simulink model "FlightController"  (R2025a)
settings: Solver=VariableStepAuto  StartTime=0.0  StopTime=10.0  RelTol=1e-3
undefined symbols (not defined in the file): K, Kt, M
libraries: slpidlib x6
settings Model: Creator=pvsha  LastModifiedBy=pvsha

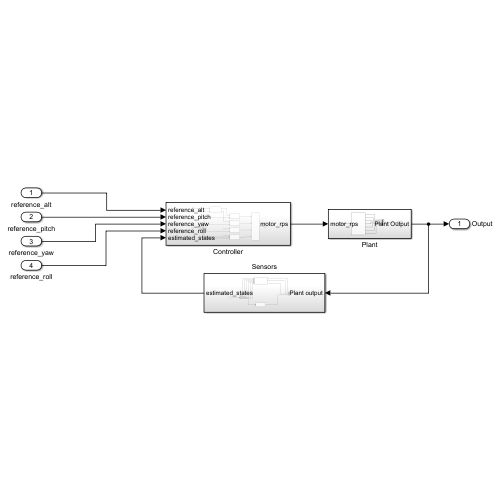
[thumbnail: Simulink's stored preview of the top-level diagram]
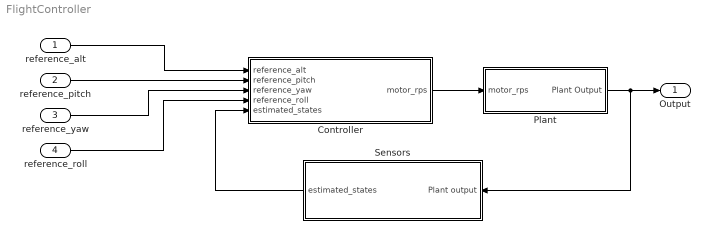
== system FlightController ==
  reference_alt : Inport
  reference_pitch : Inport  Port=2
  reference_yaw : Inport  Port=3
  reference_roll : Inport  Port=4
  Controller : Subsystem
  Plant : Subsystem
  Sensors : Subsystem
  Output : Outport  SignalName=Output
  wires:
  Controller/1(motor_rps) -> Plant/1(motor_rps)
  Sensors/1(estimated_states) -> Controller/5(estimated_states)
  Plant/1(Plant Output) -> Output/1, Sensors/1(Plant output)
  reference_alt/1 -> Controller/1(reference_alt)
  reference_pitch/1 -> Controller/2(reference_pitch)
  reference_yaw/1 -> Controller/3(reference_yaw)
  reference_roll/1 -> Controller/4(reference_roll)

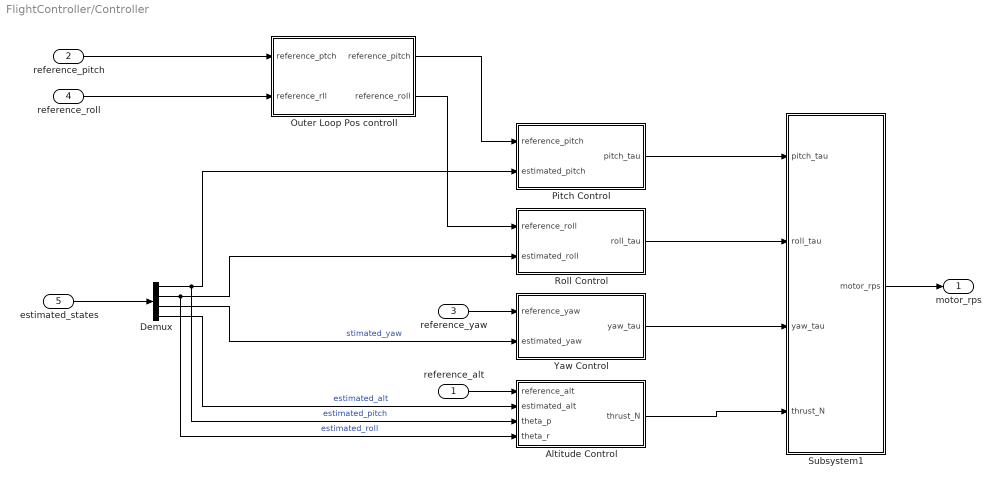
== system FlightController/Controller ==
  reference_alt : Inport
  reference_pitch : Inport  Port=2
  reference_yaw : Inport  Port=3
  reference_roll : Inport  Port=4
  estimated_states : Inport  Port=5  PortDimensions=4
  Altitude Control : Subsystem
  Demux : Demux
  Outer Loop Pos controll : Subsystem
  Pitch Control : Subsystem
  Roll Control : Subsystem
  Subsystem1 : Subsystem
  Yaw Control : Subsystem
  motor_rps : Outport
  wires:
  estimated_states/1 -> Demux/1
  Subsystem1/1(motor_rps) -> motor_rps/1
  Pitch Control/1(pitch_tau) -> Subsystem1/1(pitch_tau)
  Roll Control/1(roll_tau) -> Subsystem1/2(roll_tau)
  Altitude Control/1(thrust_N) -> Subsystem1/4(thrust_N)
  Yaw Control/1(yaw_tau) -> Subsystem1/3(yaw_tau)
  reference_yaw/1 -> Yaw Control/1(reference_yaw)
  reference_pitch/1 -> Outer Loop Pos controll/1(reference_ptch)
  reference_alt/1 -> Altitude Control/1(reference_alt)
  Demux/4 -> Altitude Control/2(estimated_alt)  "estimated_alt"
  Demux/1 -> Altitude Control/3(theta_p), Pitch Control/2(estimated_pitch)  "estimated_pitch"
  Demux/2 -> Altitude Control/4(theta_r), Roll Control/2(estimated_roll)  "estimated_roll"
  Demux/3 -> Yaw Control/2(estimated_yaw)  "stimated_yaw"
  Outer Loop Pos controll/1(reference_pitch) -> Pitch Control/1(reference_pitch)
  Outer Loop Pos controll/2(reference_roll) -> Roll Control/1(reference_roll)
  reference_roll/1 -> Outer Loop Pos controll/2(reference_rll)

== system FlightController/Plant ==
  motor_rps : Inport
  Mux : Mux  Inputs=7
  Subsystem : Subsystem
  Plant Output : Outport
  wires:
  Mux/1 -> Plant Output/1
  Subsystem/1(a_x) -> Mux/1
  Subsystem/2(a_y) -> Mux/2
  Subsystem/3(a_z) -> Mux/3
  Subsystem/4(w_p) -> Mux/4
  Subsystem/5(w_r) -> Mux/5
  Subsystem/6(w_y) -> Mux/6
  Subsystem/7(alt) -> Mux/7
  motor_rps/1 -> Subsystem/1(motor_rps)

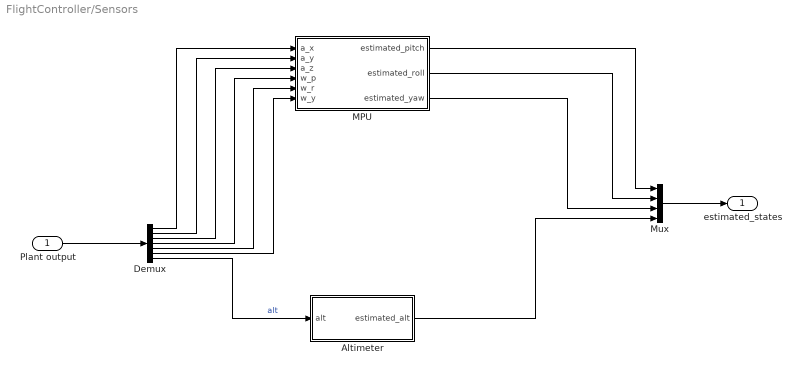
== system FlightController/Sensors ==
  Plant output : Inport
  Altimeter : Subsystem
  Demux : Demux  Outputs=7
  MPU : Subsystem
  Mux : Mux
  estimated_states : Outport
  wires:
  Plant output/1 -> Demux/1
  Demux/7 -> Altimeter/1(alt)  "alt"
  MPU/2(estimated_roll) -> Mux/2
  MPU/3(estimated_yaw) -> Mux/3
  MPU/1(estimated_pitch) -> Mux/1
  Demux/1 -> MPU/1(a_x)
  Demux/3 -> MPU/3(a_z)
  Demux/2 -> MPU/2(a_y)
  Demux/4 -> MPU/4(w_p)
  Demux/5 -> MPU/5(w_r)
  Demux/6 -> MPU/6(w_y)
  Mux/1 -> estimated_states/1
  Altimeter/1(estimated_alt) -> Mux/4

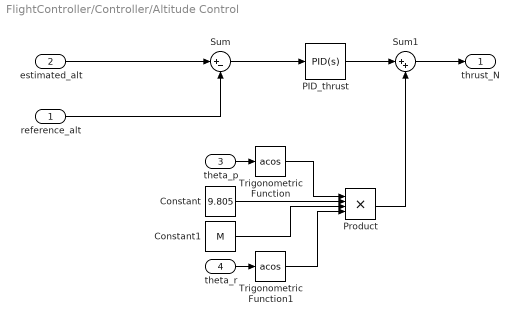
== system FlightController/Controller/Altitude Control ==
  reference_alt : Inport
  estimated_alt : Inport  Port=2
  theta_p : Inport  Port=3
  theta_r : Inport  Port=4
  Constant : Constant  Value=9.805
  Constant1 : Constant  Value=M
  PID_thrust : slpidlib/PID Controller  Controller=PID  Form=Parallel  TimeDomain=Continuous-time  UseExternalTs=off  SampleTime=-1  IntegratorMethod=Forward Euler  FilterMethod=Forward Euler  ControllerParametersSource=internal  P=1  I=1  UseKiTs=off  D=0  UseExternalDerivativeSource=off  N=100  UseFilter=on  TunerSelectOption=Transfer Function Based (PID Tuner App)  InitialConditionSource=internal  InitialConditionForIntegrator=0  InitialConditionForFilter=0  DifferentiatorICPrevScaledInput=0  ExternalReset=none  TrackingMode=off  Kt=1  LimitOutput=off  SatLimitsSource=internal  UpperSaturationLimit=inf  LowerSaturationLimit=-inf  LinearizeAsGain=on  AntiWindupMode=none  Kb=1  LimitIntegrator=off  UpperIntegratorSaturationLimit=inf  LowerIntegratorSaturationLimit=-inf  POutMin=[]  POutMax=[]  IOutMin=[]  IOutMax=[]  DOutMin=[]  DOutMax=[]  NOutMin=[]  NOutMax=[]  SumOutMin=[]  SumOutMax=[]  SaturationOutMin=[]  SaturationOutMax=[]  PParamMin=[]  PParamMax=[]  IParamMin=[]  IParamMax=[]  DParamMin=[]  DParamMax=[]  NParamMin=[]  NParamMax=[]  KbParamMin=[]  KbParamMax=[]  KtParamMin=[]  KtParamMax=[]  KbOutMin=[]  KbOutMax=[]  KtOutMin=[]  KtOutMax=[]  IntegratorOutMin=[]  IntegratorOutMax=[]  FilterOutMin=[]  FilterOutMax=[]  SumI1OutMin=[]  SumI1OutMax=[]  SumI2OutMin=[]  SumI2OutMax=[]  SumI3OutMin=[]  SumI3OutMax=[]  SumI4OutMin=[]  SumI4OutMax=[]  SumDOutMin=[]  SumDOutMax=[]  DifferentiatorOutMin=[]  DifferentiatorOutMax=[]  FilterDiffOutCoefMin=[]  FilterDiffOutCoefMax=[]  ReciprocalOutMin=[]  ReciprocalOutMax=[]  SumDenOutMin=[]  SumDenOutMax=[]  SumNumOutMin=[]  SumNumOutMax=[]  DivideOutMin=[]  DivideOutMax=[]  UdiffTsProdOutMin=[]  UdiffTsProdOutMax=[]  NTsProdOutMin=[]  NTsProdOutMax=[]  UintegralTsProdOutMin=[]  UintegralTsProdOutMax=[]  UngainTsProdOutMin=[]  UngainTsProdOutMax=[]  ClampingZeroOutDataTypeStr=Inherit: Inherit via back propagation  ClampingZeroOutMin=[]  ClampingZeroOutMax=[]  FilterDenConstantOutDataTypeStr=Inherit: Inherit via back propagation  FilterDenConstantOutMin=[]  FilterDenConstantOutMax=[]  PCopyOutDataTypeStr=Inherit: Inherit via back propagation  PCopyOutMin=[]  PCopyOutMax=[]  NCopyOutDataTypeStr=Inherit: Inherit via back propagation  NCopyOutMin=[]  NCopyOutMax=[]  IntegratorContinuousStateAttributes=''  IntegratorStateMustResolveToSignalObject=off  IntegratorRTWStateStorageClass=Auto  FilterContinuousStateAttributes=''  FilterStateMustResolveToSignalObject=off  FilterRTWStateStorageClass=Auto  ParallelPVariant=InternalParameters  IdealPVariant=Disabled  IVariant=InternalParameters  DVariant=InternalParameters  IntegratorVariant=Continuous  SatVariant=Disabled  AWVariant=Passthrough  PCopyVariant=Disabled  TRVariant=Disabled  FdbkBlocksVariant=Forward  IdealPFdbkVariant=Disabled  SatFdbkVariant=Disabled  DerivativeFilterVariant=ContFilter  NVariant=InternalParameters  NCopyVariant=Disabled  FilterICVariant=InternalICsFilter  IntegratorICVariant=InternalICs  ExternalResetVariant=Disabled  TRSumVariant=Passthrough  SumFdbkVariant=Disabled  SumVariant=Sum_PID  TsampFilterVariant=InternalTs  TsampNgainVariant=Passthrough  TsampIntegralVariant=Disabled_SignalSpec  ExternalSaturationOutDataTypeStr=Inherit: Same as second input  DerivativeSourceVariant=ErrorSignal  PreIntVariant=InternalPreInt
  Product : Product  Inputs=4
  Sum : Sum  Inputs=|+-
  Sum1 : Sum  Inputs=|++
  Trigonometric Function : Trigonometry  Operator=acos
  Trigonometric Function1 : Trigonometry  Operator=acos
  thrust_N : Outport
  wires:
  estimated_alt/1 -> Sum/1
  Sum/1 -> PID_thrust/1
  theta_p/1 -> Trigonometric Function/1
  Constant/1 -> Product/2
  Trigonometric Function/1 -> Product/1
  Constant1/1 -> Product/3
  theta_r/1 -> Trigonometric Function1/1
  Trigonometric Function1/1 -> Product/4
  reference_alt/1 -> Sum/2
  PID_thrust/1 -> Sum1/1
  Sum1/1 -> thrust_N/1
  Product/1 -> Sum1/2

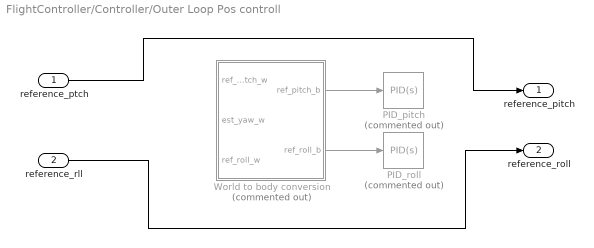
== system FlightController/Controller/Outer Loop Pos controll ==
  reference_ptch : Inport
  reference_rll : Inport  Port=2
  PID_pitch : slpidlib/PID Controller  Commented=on  Controller=PID  Form=Parallel  TimeDomain=Continuous-time  UseExternalTs=off  SampleTime=-1  IntegratorMethod=Forward Euler  FilterMethod=Forward Euler  ControllerParametersSource=internal  P=1  I=1  UseKiTs=off  D=0  UseExternalDerivativeSource=off  N=100  UseFilter=on  TunerSelectOption=Transfer Function Based (PID Tuner App)  InitialConditionSource=internal  InitialConditionForIntegrator=0  InitialConditionForFilter=0  DifferentiatorICPrevScaledInput=0  ExternalReset=none  TrackingMode=off  Kt=1  LimitOutput=off  SatLimitsSource=internal  UpperSaturationLimit=inf  LowerSaturationLimit=-inf  LinearizeAsGain=on  AntiWindupMode=none  Kb=1  LimitIntegrator=off  UpperIntegratorSaturationLimit=inf  LowerIntegratorSaturationLimit=-inf  POutMin=[]  POutMax=[]  IOutMin=[]  IOutMax=[]  DOutMin=[]  DOutMax=[]  NOutMin=[]  NOutMax=[]  SumOutMin=[]  SumOutMax=[]  SaturationOutMin=[]  SaturationOutMax=[]  PParamMin=[]  PParamMax=[]  IParamMin=[]  IParamMax=[]  DParamMin=[]  DParamMax=[]  NParamMin=[]  NParamMax=[]  KbParamMin=[]  KbParamMax=[]  KtParamMin=[]  KtParamMax=[]  KbOutMin=[]  KbOutMax=[]  KtOutMin=[]  KtOutMax=[]  IntegratorOutMin=[]  IntegratorOutMax=[]  FilterOutMin=[]  FilterOutMax=[]  SumI1OutMin=[]  SumI1OutMax=[]  SumI2OutMin=[]  SumI2OutMax=[]  SumI3OutMin=[]  SumI3OutMax=[]  SumI4OutMin=[]  SumI4OutMax=[]  SumDOutMin=[]  SumDOutMax=[]  DifferentiatorOutMin=[]  DifferentiatorOutMax=[]  FilterDiffOutCoefMin=[]  FilterDiffOutCoefMax=[]  ReciprocalOutMin=[]  ReciprocalOutMax=[]  SumDenOutMin=[]  SumDenOutMax=[]  SumNumOutMin=[]  SumNumOutMax=[]  DivideOutMin=[]  DivideOutMax=[]  UdiffTsProdOutMin=[]  UdiffTsProdOutMax=[]  NTsProdOutMin=[]  NTsProdOutMax=[]  UintegralTsProdOutMin=[]  UintegralTsProdOutMax=[]  UngainTsProdOutMin=[]  UngainTsProdOutMax=[]  ClampingZeroOutDataTypeStr=Inherit: Inherit via back propagation  ClampingZeroOutMin=[]  ClampingZeroOutMax=[]  FilterDenConstantOutDataTypeStr=Inherit: Inherit via back propagation  FilterDenConstantOutMin=[]  FilterDenConstantOutMax=[]  PCopyOutDataTypeStr=Inherit: Inherit via back propagation  PCopyOutMin=[]  PCopyOutMax=[]  NCopyOutDataTypeStr=Inherit: Inherit via back propagation  NCopyOutMin=[]  NCopyOutMax=[]  IntegratorContinuousStateAttributes=''  IntegratorStateMustResolveToSignalObject=off  IntegratorRTWStateStorageClass=Auto  FilterContinuousStateAttributes=''  FilterStateMustResolveToSignalObject=off  FilterRTWStateStorageClass=Auto  ParallelPVariant=InternalParameters  IdealPVariant=Disabled  IVariant=InternalParameters  DVariant=InternalParameters  IntegratorVariant=Continuous  SatVariant=Disabled  AWVariant=Passthrough  PCopyVariant=Disabled  TRVariant=Disabled  FdbkBlocksVariant=Forward  IdealPFdbkVariant=Disabled  SatFdbkVariant=Disabled  DerivativeFilterVariant=ContFilter  NVariant=InternalParameters  NCopyVariant=Disabled  FilterICVariant=InternalICsFilter  IntegratorICVariant=InternalICs  ExternalResetVariant=Disabled  TRSumVariant=Passthrough  SumFdbkVariant=Disabled  SumVariant=Sum_PID  TsampFilterVariant=InternalTs  TsampNgainVariant=Passthrough  TsampIntegralVariant=Disabled_SignalSpec  ExternalSaturationOutDataTypeStr=Inherit: Same as second input  DerivativeSourceVariant=ErrorSignal  PreIntVariant=InternalPreInt
  PID_roll : slpidlib/PID Controller  Commented=on  Controller=PID  Form=Parallel  TimeDomain=Continuous-time  UseExternalTs=off  SampleTime=-1  IntegratorMethod=Forward Euler  FilterMethod=Forward Euler  ControllerParametersSource=internal  P=1  I=1  UseKiTs=off  D=0  UseExternalDerivativeSource=off  N=100  UseFilter=on  TunerSelectOption=Transfer Function Based (PID Tuner App)  InitialConditionSource=internal  InitialConditionForIntegrator=0  InitialConditionForFilter=0  DifferentiatorICPrevScaledInput=0  ExternalReset=none  TrackingMode=off  Kt=1  LimitOutput=off  SatLimitsSource=internal  UpperSaturationLimit=inf  LowerSaturationLimit=-inf  LinearizeAsGain=on  AntiWindupMode=none  Kb=1  LimitIntegrator=off  UpperIntegratorSaturationLimit=inf  LowerIntegratorSaturationLimit=-inf  POutMin=[]  POutMax=[]  IOutMin=[]  IOutMax=[]  DOutMin=[]  DOutMax=[]  NOutMin=[]  NOutMax=[]  SumOutMin=[]  SumOutMax=[]  SaturationOutMin=[]  SaturationOutMax=[]  PParamMin=[]  PParamMax=[]  IParamMin=[]  IParamMax=[]  DParamMin=[]  DParamMax=[]  NParamMin=[]  NParamMax=[]  KbParamMin=[]  KbParamMax=[]  KtParamMin=[]  KtParamMax=[]  KbOutMin=[]  KbOutMax=[]  KtOutMin=[]  KtOutMax=[]  IntegratorOutMin=[]  IntegratorOutMax=[]  FilterOutMin=[]  FilterOutMax=[]  SumI1OutMin=[]  SumI1OutMax=[]  SumI2OutMin=[]  SumI2OutMax=[]  SumI3OutMin=[]  SumI3OutMax=[]  SumI4OutMin=[]  SumI4OutMax=[]  SumDOutMin=[]  SumDOutMax=[]  DifferentiatorOutMin=[]  DifferentiatorOutMax=[]  FilterDiffOutCoefMin=[]  FilterDiffOutCoefMax=[]  ReciprocalOutMin=[]  ReciprocalOutMax=[]  SumDenOutMin=[]  SumDenOutMax=[]  SumNumOutMin=[]  SumNumOutMax=[]  DivideOutMin=[]  DivideOutMax=[]  UdiffTsProdOutMin=[]  UdiffTsProdOutMax=[]  NTsProdOutMin=[]  NTsProdOutMax=[]  UintegralTsProdOutMin=[]  UintegralTsProdOutMax=[]  UngainTsProdOutMin=[]  UngainTsProdOutMax=[]  ClampingZeroOutDataTypeStr=Inherit: Inherit via back propagation  ClampingZeroOutMin=[]  ClampingZeroOutMax=[]  FilterDenConstantOutDataTypeStr=Inherit: Inherit via back propagation  FilterDenConstantOutMin=[]  FilterDenConstantOutMax=[]  PCopyOutDataTypeStr=Inherit: Inherit via back propagation  PCopyOutMin=[]  PCopyOutMax=[]  NCopyOutDataTypeStr=Inherit: Inherit via back propagation  NCopyOutMin=[]  NCopyOutMax=[]  IntegratorContinuousStateAttributes=''  IntegratorStateMustResolveToSignalObject=off  IntegratorRTWStateStorageClass=Auto  FilterContinuousStateAttributes=''  FilterStateMustResolveToSignalObject=off  FilterRTWStateStorageClass=Auto  ParallelPVariant=InternalParameters  IdealPVariant=Disabled  IVariant=InternalParameters  DVariant=InternalParameters  IntegratorVariant=Continuous  SatVariant=Disabled  AWVariant=Passthrough  PCopyVariant=Disabled  TRVariant=Disabled  FdbkBlocksVariant=Forward  IdealPFdbkVariant=Disabled  SatFdbkVariant=Disabled  DerivativeFilterVariant=ContFilter  NVariant=InternalParameters  NCopyVariant=Disabled  FilterICVariant=InternalICsFilter  IntegratorICVariant=InternalICs  ExternalResetVariant=Disabled  TRSumVariant=Passthrough  SumFdbkVariant=Disabled  SumVariant=Sum_PID  TsampFilterVariant=InternalTs  TsampNgainVariant=Passthrough  TsampIntegralVariant=Disabled_SignalSpec  ExternalSaturationOutDataTypeStr=Inherit: Same as second input  DerivativeSourceVariant=ErrorSignal  PreIntVariant=InternalPreInt
  World to body conversion : Subsystem  Commented=on
  reference_pitch : Outport
  reference_roll : Outport  Port=2
  wires:
  World to body conversion/1(ref_pitch_b) -> PID_pitch/1
  World to body conversion/2(ref_roll_b) -> PID_roll/1
  reference_ptch/1 -> reference_pitch/1
  reference_rll/1 -> reference_roll/1

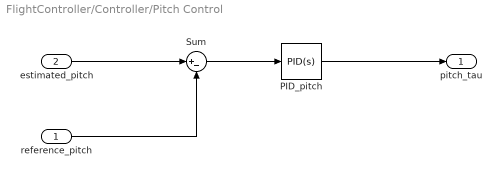
== system FlightController/Controller/Pitch Control ==
  reference_pitch : Inport
  estimated_pitch : Inport  Port=2
  PID_pitch : slpidlib/PID Controller  Controller=PID  Form=Parallel  TimeDomain=Continuous-time  UseExternalTs=off  SampleTime=-1  IntegratorMethod=Forward Euler  FilterMethod=Forward Euler  ControllerParametersSource=internal  P=1  I=1  UseKiTs=off  D=0  UseExternalDerivativeSource=off  N=100  UseFilter=on  TunerSelectOption=Transfer Function Based (PID Tuner App)  InitialConditionSource=internal  InitialConditionForIntegrator=0  InitialConditionForFilter=0  DifferentiatorICPrevScaledInput=0  ExternalReset=none  TrackingMode=off  Kt=1  LimitOutput=off  SatLimitsSource=internal  UpperSaturationLimit=inf  LowerSaturationLimit=-inf  LinearizeAsGain=on  AntiWindupMode=none  Kb=1  LimitIntegrator=off  UpperIntegratorSaturationLimit=inf  LowerIntegratorSaturationLimit=-inf  POutMin=[]  POutMax=[]  IOutMin=[]  IOutMax=[]  DOutMin=[]  DOutMax=[]  NOutMin=[]  NOutMax=[]  SumOutMin=[]  SumOutMax=[]  SaturationOutMin=[]  SaturationOutMax=[]  PParamMin=[]  PParamMax=[]  IParamMin=[]  IParamMax=[]  DParamMin=[]  DParamMax=[]  NParamMin=[]  NParamMax=[]  KbParamMin=[]  KbParamMax=[]  KtParamMin=[]  KtParamMax=[]  KbOutMin=[]  KbOutMax=[]  KtOutMin=[]  KtOutMax=[]  IntegratorOutMin=[]  IntegratorOutMax=[]  FilterOutMin=[]  FilterOutMax=[]  SumI1OutMin=[]  SumI1OutMax=[]  SumI2OutMin=[]  SumI2OutMax=[]  SumI3OutMin=[]  SumI3OutMax=[]  SumI4OutMin=[]  SumI4OutMax=[]  SumDOutMin=[]  SumDOutMax=[]  DifferentiatorOutMin=[]  DifferentiatorOutMax=[]  FilterDiffOutCoefMin=[]  FilterDiffOutCoefMax=[]  ReciprocalOutMin=[]  ReciprocalOutMax=[]  SumDenOutMin=[]  SumDenOutMax=[]  SumNumOutMin=[]  SumNumOutMax=[]  DivideOutMin=[]  DivideOutMax=[]  UdiffTsProdOutMin=[]  UdiffTsProdOutMax=[]  NTsProdOutMin=[]  NTsProdOutMax=[]  UintegralTsProdOutMin=[]  UintegralTsProdOutMax=[]  UngainTsProdOutMin=[]  UngainTsProdOutMax=[]  ClampingZeroOutDataTypeStr=Inherit: Inherit via back propagation  ClampingZeroOutMin=[]  ClampingZeroOutMax=[]  FilterDenConstantOutDataTypeStr=Inherit: Inherit via back propagation  FilterDenConstantOutMin=[]  FilterDenConstantOutMax=[]  PCopyOutDataTypeStr=Inherit: Inherit via back propagation  PCopyOutMin=[]  PCopyOutMax=[]  NCopyOutDataTypeStr=Inherit: Inherit via back propagation  NCopyOutMin=[]  NCopyOutMax=[]  IntegratorContinuousStateAttributes=''  IntegratorStateMustResolveToSignalObject=off  IntegratorRTWStateStorageClass=Auto  FilterContinuousStateAttributes=''  FilterStateMustResolveToSignalObject=off  FilterRTWStateStorageClass=Auto  ParallelPVariant=InternalParameters  IdealPVariant=Disabled  IVariant=InternalParameters  DVariant=InternalParameters  IntegratorVariant=Continuous  SatVariant=Disabled  AWVariant=Passthrough  PCopyVariant=Disabled  TRVariant=Disabled  FdbkBlocksVariant=Forward  IdealPFdbkVariant=Disabled  SatFdbkVariant=Disabled  DerivativeFilterVariant=ContFilter  NVariant=InternalParameters  NCopyVariant=Disabled  FilterICVariant=InternalICsFilter  IntegratorICVariant=InternalICs  ExternalResetVariant=Disabled  TRSumVariant=Passthrough  SumFdbkVariant=Disabled  SumVariant=Sum_PID  TsampFilterVariant=InternalTs  TsampNgainVariant=Passthrough  TsampIntegralVariant=Disabled_SignalSpec  ExternalSaturationOutDataTypeStr=Inherit: Same as second input  DerivativeSourceVariant=ErrorSignal  PreIntVariant=InternalPreInt
  Sum : Sum  Inputs=|+-
  pitch_tau : Outport
  wires:
  estimated_pitch/1 -> Sum/1
  reference_pitch/1 -> Sum/2
  Sum/1 -> PID_pitch/1
  PID_pitch/1 -> pitch_tau/1

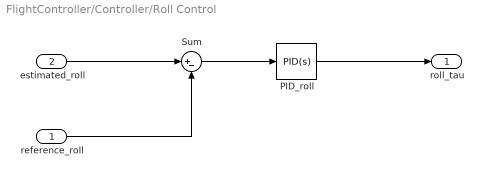
== system FlightController/Controller/Roll Control ==
  reference_roll : Inport
  estimated_roll : Inport  Port=2
  PID_roll : slpidlib/PID Controller  Controller=PID  Form=Parallel  TimeDomain=Continuous-time  UseExternalTs=off  SampleTime=-1  IntegratorMethod=Forward Euler  FilterMethod=Forward Euler  ControllerParametersSource=internal  P=1  I=1  UseKiTs=off  D=0  UseExternalDerivativeSource=off  N=100  UseFilter=on  TunerSelectOption=Transfer Function Based (PID Tuner App)  InitialConditionSource=internal  InitialConditionForIntegrator=0  InitialConditionForFilter=0  DifferentiatorICPrevScaledInput=0  ExternalReset=none  TrackingMode=off  Kt=1  LimitOutput=off  SatLimitsSource=internal  UpperSaturationLimit=inf  LowerSaturationLimit=-inf  LinearizeAsGain=on  AntiWindupMode=none  Kb=1  LimitIntegrator=off  UpperIntegratorSaturationLimit=inf  LowerIntegratorSaturationLimit=-inf  POutMin=[]  POutMax=[]  IOutMin=[]  IOutMax=[]  DOutMin=[]  DOutMax=[]  NOutMin=[]  NOutMax=[]  SumOutMin=[]  SumOutMax=[]  SaturationOutMin=[]  SaturationOutMax=[]  PParamMin=[]  PParamMax=[]  IParamMin=[]  IParamMax=[]  DParamMin=[]  DParamMax=[]  NParamMin=[]  NParamMax=[]  KbParamMin=[]  KbParamMax=[]  KtParamMin=[]  KtParamMax=[]  KbOutMin=[]  KbOutMax=[]  KtOutMin=[]  KtOutMax=[]  IntegratorOutMin=[]  IntegratorOutMax=[]  FilterOutMin=[]  FilterOutMax=[]  SumI1OutMin=[]  SumI1OutMax=[]  SumI2OutMin=[]  SumI2OutMax=[]  SumI3OutMin=[]  SumI3OutMax=[]  SumI4OutMin=[]  SumI4OutMax=[]  SumDOutMin=[]  SumDOutMax=[]  DifferentiatorOutMin=[]  DifferentiatorOutMax=[]  FilterDiffOutCoefMin=[]  FilterDiffOutCoefMax=[]  ReciprocalOutMin=[]  ReciprocalOutMax=[]  SumDenOutMin=[]  SumDenOutMax=[]  SumNumOutMin=[]  SumNumOutMax=[]  DivideOutMin=[]  DivideOutMax=[]  UdiffTsProdOutMin=[]  UdiffTsProdOutMax=[]  NTsProdOutMin=[]  NTsProdOutMax=[]  UintegralTsProdOutMin=[]  UintegralTsProdOutMax=[]  UngainTsProdOutMin=[]  UngainTsProdOutMax=[]  ClampingZeroOutDataTypeStr=Inherit: Inherit via back propagation  ClampingZeroOutMin=[]  ClampingZeroOutMax=[]  FilterDenConstantOutDataTypeStr=Inherit: Inherit via back propagation  FilterDenConstantOutMin=[]  FilterDenConstantOutMax=[]  PCopyOutDataTypeStr=Inherit: Inherit via back propagation  PCopyOutMin=[]  PCopyOutMax=[]  NCopyOutDataTypeStr=Inherit: Inherit via back propagation  NCopyOutMin=[]  NCopyOutMax=[]  IntegratorContinuousStateAttributes=''  IntegratorStateMustResolveToSignalObject=off  IntegratorRTWStateStorageClass=Auto  FilterContinuousStateAttributes=''  FilterStateMustResolveToSignalObject=off  FilterRTWStateStorageClass=Auto  ParallelPVariant=InternalParameters  IdealPVariant=Disabled  IVariant=InternalParameters  DVariant=InternalParameters  IntegratorVariant=Continuous  SatVariant=Disabled  AWVariant=Passthrough  PCopyVariant=Disabled  TRVariant=Disabled  FdbkBlocksVariant=Forward  IdealPFdbkVariant=Disabled  SatFdbkVariant=Disabled  DerivativeFilterVariant=ContFilter  NVariant=InternalParameters  NCopyVariant=Disabled  FilterICVariant=InternalICsFilter  IntegratorICVariant=InternalICs  ExternalResetVariant=Disabled  TRSumVariant=Passthrough  SumFdbkVariant=Disabled  SumVariant=Sum_PID  TsampFilterVariant=InternalTs  TsampNgainVariant=Passthrough  TsampIntegralVariant=Disabled_SignalSpec  ExternalSaturationOutDataTypeStr=Inherit: Same as second input  DerivativeSourceVariant=ErrorSignal  PreIntVariant=InternalPreInt
  Sum : Sum  Inputs=|+-
  roll_tau : Outport
  wires:
  estimated_roll/1 -> Sum/1
  PID_roll/1 -> roll_tau/1
  reference_roll/1 -> Sum/2
  Sum/1 -> PID_roll/1

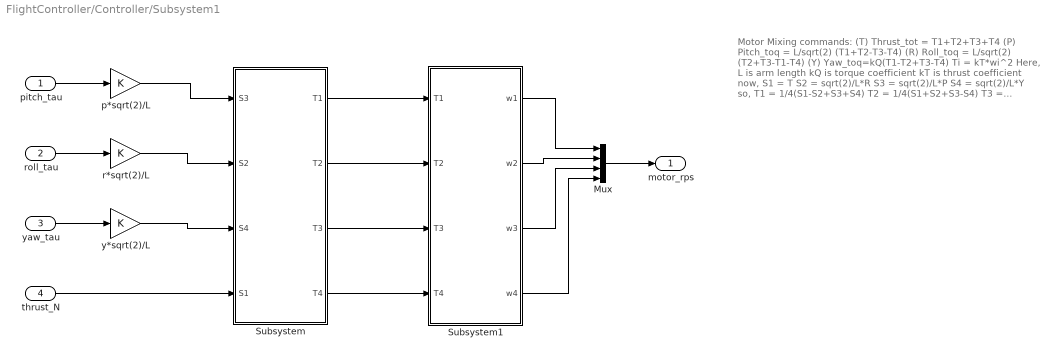
== system FlightController/Controller/Subsystem1 ==
  note: Motor Mixing commands:
      |
      | (T) Thrust_tot = T1+T2+T3+T4
      | (P) Pitch_toq = L/sqrt(2) (T1+T2-T3-T4)
      | (R) Roll_toq = L/sqrt(2) (T2+T3-T1-T4)
      | (Y) Yaw_toq=kQ(T1-T2+T3-T4)
      | Ti = kT*wi^2
      |
      | Here,
      | L is arm length
      | kQ is torque coefficient
      | kT is thrust coefficient
      |
      | now,
      | S1 = T
      | S2 = sqrt(2)/L*R
      | S3 = sqrt(2)/L*P
      | S4 = sqrt(2)/L*Y
      |
      | so,
      | T1 = 1/4(S1-S2+S3+S4)
      | T2 = 1/4(S1+S2+S3-S4)
      | T3 = 1/4(S1+S2-S3+S4)
      | T4 = 1/4(S1-S2-S3-S4)
      |
      | and ofcourse,
      | wi = sqrt(Ti/kT)
  pitch_tau : Inport
  roll_tau : Inport  Port=2
  yaw_tau : Inport  Port=3
  thrust_N : Inport  Port=4
  Mux : Mux
  Subsystem : Subsystem
  Subsystem1 : Subsystem
  p*sqrt(2)/L : Gain  Gain=K
  r*sqrt(2)/L : Gain  Gain=K
  y*sqrt(2)/L : Gain  Gain=K
  motor_rps : Outport
  wires:
  pitch_tau/1 -> p*sqrt(2)/L/1
  roll_tau/1 -> r*sqrt(2)/L/1
  yaw_tau/1 -> y*sqrt(2)/L/1
  p*sqrt(2)/L/1 -> Subsystem/1(S3)
  r*sqrt(2)/L/1 -> Subsystem/2(S2)
  y*sqrt(2)/L/1 -> Subsystem/3(S4)
  thrust_N/1 -> Subsystem/4(S1)
  Subsystem/1(T1) -> Subsystem1/1(T1)
  Subsystem/2(T2) -> Subsystem1/2(T2)
  Subsystem/3(T3) -> Subsystem1/3(T3)
  Subsystem/4(T4) -> Subsystem1/4(T4)
  Subsystem1/1(w1) -> Mux/1
  Subsystem1/2(w2) -> Mux/2
  Subsystem1/3(w3) -> Mux/3
  Subsystem1/4(w4) -> Mux/4
  Mux/1 -> motor_rps/1

== system FlightController/Controller/Yaw Control ==
  reference_yaw : Inport
  estimated_yaw : Inport  Port=2
  PID_yaw : slpidlib/PID Controller  Controller=PID  Form=Parallel  TimeDomain=Continuous-time  UseExternalTs=off  SampleTime=-1  IntegratorMethod=Forward Euler  FilterMethod=Forward Euler  ControllerParametersSource=internal  P=1  I=1  UseKiTs=off  D=0  UseExternalDerivativeSource=off  N=100  UseFilter=on  TunerSelectOption=Transfer Function Based (PID Tuner App)  InitialConditionSource=internal  InitialConditionForIntegrator=0  InitialConditionForFilter=0  DifferentiatorICPrevScaledInput=0  ExternalReset=none  TrackingMode=off  Kt=1  LimitOutput=off  SatLimitsSource=internal  UpperSaturationLimit=inf  LowerSaturationLimit=-inf  LinearizeAsGain=on  AntiWindupMode=none  Kb=1  LimitIntegrator=off  UpperIntegratorSaturationLimit=inf  LowerIntegratorSaturationLimit=-inf  POutMin=[]  POutMax=[]  IOutMin=[]  IOutMax=[]  DOutMin=[]  DOutMax=[]  NOutMin=[]  NOutMax=[]  SumOutMin=[]  SumOutMax=[]  SaturationOutMin=[]  SaturationOutMax=[]  PParamMin=[]  PParamMax=[]  IParamMin=[]  IParamMax=[]  DParamMin=[]  DParamMax=[]  NParamMin=[]  NParamMax=[]  KbParamMin=[]  KbParamMax=[]  KtParamMin=[]  KtParamMax=[]  KbOutMin=[]  KbOutMax=[]  KtOutMin=[]  KtOutMax=[]  IntegratorOutMin=[]  IntegratorOutMax=[]  FilterOutMin=[]  FilterOutMax=[]  SumI1OutMin=[]  SumI1OutMax=[]  SumI2OutMin=[]  SumI2OutMax=[]  SumI3OutMin=[]  SumI3OutMax=[]  SumI4OutMin=[]  SumI4OutMax=[]  SumDOutMin=[]  SumDOutMax=[]  DifferentiatorOutMin=[]  DifferentiatorOutMax=[]  FilterDiffOutCoefMin=[]  FilterDiffOutCoefMax=[]  ReciprocalOutMin=[]  ReciprocalOutMax=[]  SumDenOutMin=[]  SumDenOutMax=[]  SumNumOutMin=[]  SumNumOutMax=[]  DivideOutMin=[]  DivideOutMax=[]  UdiffTsProdOutMin=[]  UdiffTsProdOutMax=[]  NTsProdOutMin=[]  NTsProdOutMax=[]  UintegralTsProdOutMin=[]  UintegralTsProdOutMax=[]  UngainTsProdOutMin=[]  UngainTsProdOutMax=[]  ClampingZeroOutDataTypeStr=Inherit: Inherit via back propagation  ClampingZeroOutMin=[]  ClampingZeroOutMax=[]  FilterDenConstantOutDataTypeStr=Inherit: Inherit via back propagation  FilterDenConstantOutMin=[]  FilterDenConstantOutMax=[]  PCopyOutDataTypeStr=Inherit: Inherit via back propagation  PCopyOutMin=[]  PCopyOutMax=[]  NCopyOutDataTypeStr=Inherit: Inherit via back propagation  NCopyOutMin=[]  NCopyOutMax=[]  IntegratorContinuousStateAttributes=''  IntegratorStateMustResolveToSignalObject=off  IntegratorRTWStateStorageClass=Auto  FilterContinuousStateAttributes=''  FilterStateMustResolveToSignalObject=off  FilterRTWStateStorageClass=Auto  ParallelPVariant=InternalParameters  IdealPVariant=Disabled  IVariant=InternalParameters  DVariant=InternalParameters  IntegratorVariant=Continuous  SatVariant=Disabled  AWVariant=Passthrough  PCopyVariant=Disabled  TRVariant=Disabled  FdbkBlocksVariant=Forward  IdealPFdbkVariant=Disabled  SatFdbkVariant=Disabled  DerivativeFilterVariant=ContFilter  NVariant=InternalParameters  NCopyVariant=Disabled  FilterICVariant=InternalICsFilter  IntegratorICVariant=InternalICs  ExternalResetVariant=Disabled  TRSumVariant=Passthrough  SumFdbkVariant=Disabled  SumVariant=Sum_PID  TsampFilterVariant=InternalTs  TsampNgainVariant=Passthrough  TsampIntegralVariant=Disabled_SignalSpec  ExternalSaturationOutDataTypeStr=Inherit: Same as second input  DerivativeSourceVariant=ErrorSignal  PreIntVariant=InternalPreInt
  Sum : Sum  Inputs=|+-
  yaw_tau : Outport
  wires:
  estimated_yaw/1 -> Sum/1
  PID_yaw/1 -> yaw_tau/1
  reference_yaw/1 -> Sum/2
  Sum/1 -> PID_yaw/1

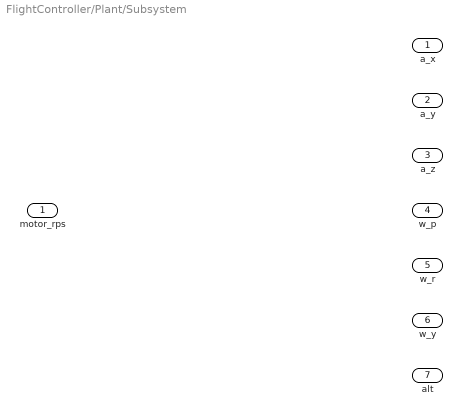
== system FlightController/Plant/Subsystem ==
  motor_rps : Inport
  a_x : Outport
  a_y : Outport  Port=2
  a_z : Outport  Port=3
  w_p : Outport  Port=4
  w_r : Outport  Port=5
  w_y : Outport  Port=6
  alt : Outport  Port=7

== system FlightController/Sensors/Altimeter ==
  alt : Inport
  estimated_alt : Outport

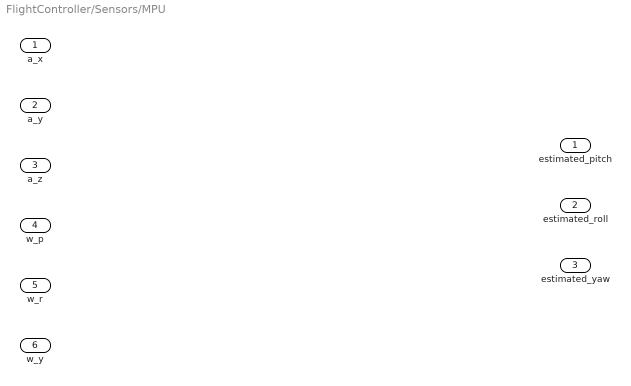
== system FlightController/Sensors/MPU ==
  a_x : Inport
  a_y : Inport  Port=2
  a_z : Inport  Port=3
  w_p : Inport  Port=4
  w_r : Inport  Port=5
  w_y : Inport  Port=6
  estimated_pitch : Outport
  estimated_roll : Outport  Port=2
  estimated_yaw : Outport  Port=3

== system FlightController/Controller/Outer Loop Pos controll/World to body conversion ==
  ref_pitch_w : Inport
  est_yaw_w : Inport  Port=2
  ref_roll_w : Inport  Port=3
  ref_pitch_b : Outport
  ref_roll_b : Outport  Port=2

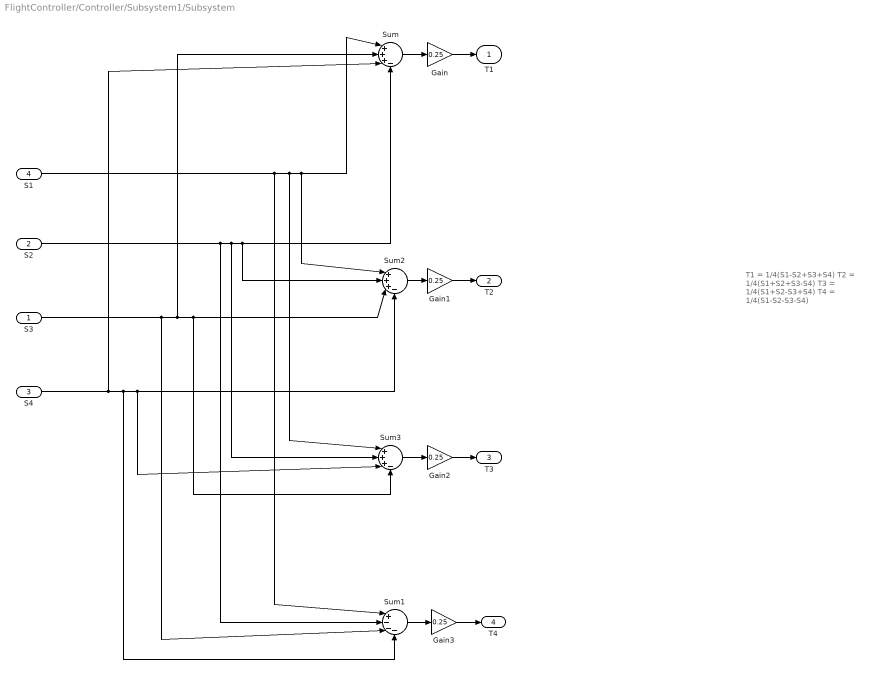
== system FlightController/Controller/Subsystem1/Subsystem ==
  note: T1 = 1/4(S1-S2+S3+S4)
      | T2 = 1/4(S1+S2+S3-S4)
      | T3 = 1/4(S1+S2-S3+S4)
      | T4 = 1/4(S1-S2-S3-S4)
  S3 : Inport
  S2 : Inport  Port=2
  S4 : Inport  Port=3
  S1 : Inport  Port=4
  Gain{,1..3} (4 alike) : Gain  Gain=0.25
  Sum : Sum  Inputs=|+++-
  Sum1 : Sum  Inputs=|+---
  Sum2 : Sum  Inputs=|+++-
  Sum3 : Sum  Inputs=|+++-
  T1 : Outport
  T2 : Outport  Port=2
  T3 : Outport  Port=3
  T4 : Outport  Port=4
  wires:
  Gain3/1 -> T4/1
  Gain2/1 -> T3/1
  Gain1/1 -> T2/1
  Gain/1 -> T1/1
  S1/1 -> Sum/1, Sum2/1, Sum3/1, Sum1/1
  S3/1 -> Sum3/4, Sum2/3, Sum/2, Sum1/3
  S4/1 -> Sum2/4, Sum3/3, Sum1/4, Sum/3
  S2/1 -> Sum1/2, Sum2/2, Sum/4, Sum3/2
  Sum/1 -> Gain/1
  Sum3/1 -> Gain2/1
  Sum2/1 -> Gain1/1
  Sum1/1 -> Gain3/1

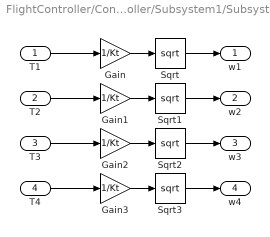
== system FlightController/Controller/Subsystem1/Subsystem1 ==
  T1 : Inport
  T2 : Inport  Port=2
  T3 : Inport  Port=3
  T4 : Inport  Port=4
  Gain{,1..3} (4 alike) : Gain  Gain=1/Kt
  Sqrt{,1..3} (4 alike) : Sqrt
  w1 : Outport
  w2 : Outport  Port=2
  w3 : Outport  Port=3
  w4 : Outport  Port=4
  wires:
  T1/1 -> Gain/1
  T2/1 -> Gain1/1
  T3/1 -> Gain2/1
  T4/1 -> Gain3/1
  Gain3/1 -> Sqrt3/1
  Gain2/1 -> Sqrt2/1
  Gain/1 -> Sqrt/1
  Gain1/1 -> Sqrt1/1
  Sqrt/1 -> w1/1
  Sqrt1/1 -> w2/1
  Sqrt2/1 -> w3/1
  Sqrt3/1 -> w4/1
